simulink model "simulinkExemplo"  (R2021a)
settings: Solver=VariableStepAuto  StartTime=0.0  StopTime=10.0  RelTol=1e-3
libraries: simulink x1
settings Model: Creator=Pedrus  LastModifiedBy=Pedrus

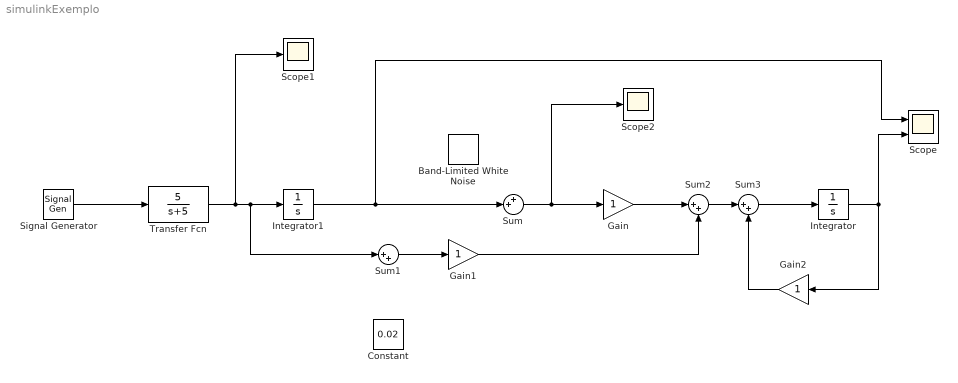
== system simulinkExemplo ==
  Band-Limited White Noise : simulink/Sources/Band-Limited White Noise  Cov=[0.1]  Ts=0.1  seed=[23341]
  Constant : Constant  Value=0.02
  Gain : Gain
  Gain1 : Gain
  Gain2 : Gain
  Integrator : Integrator
  Integrator1 : Integrator
  Scope : Scope  NumInputPorts=2
  Scope1 : Scope
  Scope2 : Scope
  Signal Generator : SignalGenerator  WaveForm=square  Units=rad/sec
  Sum : Sum  Inputs=++|
  Sum1 : Sum  Inputs=|++
  Sum2 : Sum  Inputs=|++
  Sum3 : Sum  Inputs=|++
  Transfer Fcn : TransferFcn  Numerator=[5]  Denominator=[1 5]
  wires:
  Transfer Fcn/1 -> Scope1/1, Sum1/1, Integrator1/1
  Signal Generator/1 -> Transfer Fcn/1
  Integrator1/1 -> Scope/1, Sum/2
  Sum1/1 -> Gain1/1
  Sum2/1 -> Sum3/1
  Sum/1 -> Scope2/1, Gain/1
  Gain/1 -> Sum2/1
  Gain2/1 -> Sum3/2
  Integrator/1 -> Scope/2, Gain2/1
  Sum3/1 -> Integrator/1
  Gain1/1 -> Sum2/2
